simulink model "mrsMultiRobotAvoidance"  (R2019b)
settings: Solver=FixedStepAuto  StartTime=0.0  StopTime=inf  FixedStep=sampleTime  RelTol=1e-3
PreLoadFcn:
  | % Simulation parameters
  | load exampleMap
  | sampleTime = 0.05;
  | 
  | % Robot parameters
  | wheelRadius = 0.025;
  | robotRadius = 0.35;
  | 
  | % Lidar parameters
  | sensorOffset = [0,0];
  | scanAngles = linspace(-pi/2,pi/2,9)';
  | maxRange = 5;
libraries: mobileRoboticsLib x4
settings Model: EnablePacing=on  Creator=scastro  LastModifiedBy=jayas
settings DataIOCC: ReturnWorkspaceOutputs=off
settings DebuggingCC: PregeneratedLibrarySubsystemCodeDiagnostic=none  ArithmeticOperatorsInVariantConditions=warning
settings SFSimCC: SimUseLocalCustomCode=off  CustomCodeUndefinedFunction=UseInterfaceOnly
settings RTWCC: RTWUseLocalCustomCode=off

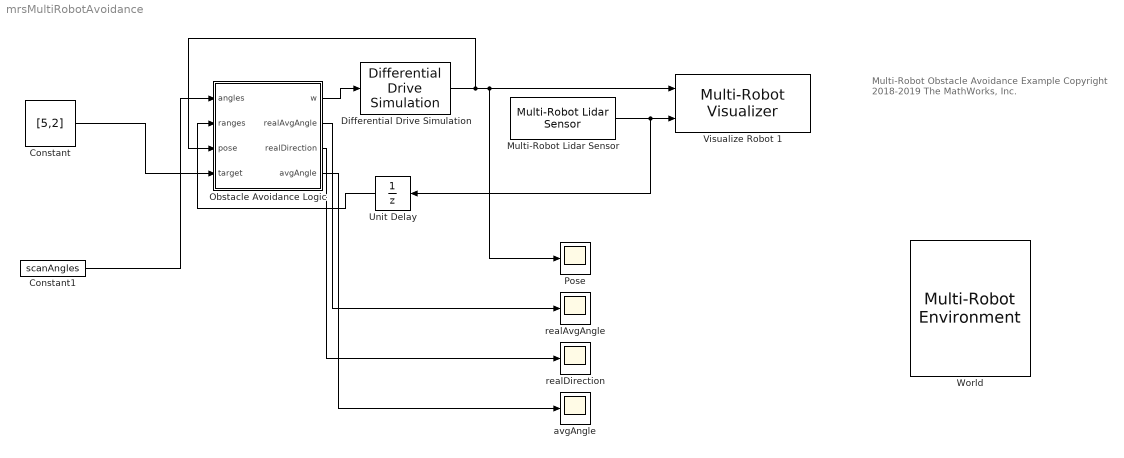
== system mrsMultiRobotAvoidance ==
  note: Multi-Robot Obstacle
      | Avoidance Example
      |
      | Copyright 2018-2019 The MathWorks, Inc.
  Constant : Constant  Value=[5,2]
  Constant1 : Constant  Value=scanAngles
  Differential Drive Simulation : mobileRoboticsLib/Kinematic Models/Differential Drive/Differential Drive Simulation  wheelRadius=wheelRadius  wheelBase=robotRadius  initX=10  initY=10  initAngle=0  Ts=sampleTime
      settings: SourceProductName=Mobile Robotics Simulation Toolbox
  Multi-Robot Lidar Sensor : mobileRoboticsLib/Environments/Multi-Robot Lidar Sensor  robotIdx=1  mapName=map  sensorOffset=sensorOffset  scanAngles=scanAngles  maxRange=maxRange
      settings: SourceProductName=Mobile Robotics Simulation Toolbox
  Obstacle Avoidance Logic : Stateflow chart  TreatAsAtomicUnit=on
  Pose : Scope
  Unit Delay : UnitDelay  SampleTime=-1  HasFrameUpgradeWarning=on
  Visualize Robot 1 : mobileRoboticsLib/Environments/Multi-Robot Visualizer  idx=1  radius=robotRadius  robotColor=[0 0 1]  showTraj=off  hasLidar=on  sensorOffset=sensorOffset  scanAngles=scanAngles  maxNumScans=0  hasObjDetector=off  objDetectorOffset=[0,0]  objDetectorAngle=0  objDetectorFOV=pi/2  objDetectorMaxRange=5  hasRobotDetector=off  robotDetectorOffset=[0,0]  robotDetectorAngle=0  robotDetectorFOV=pi/3  robotDetectorMaxRange=5  robotDetectorNumDetections=0
      settings: SourceProductName=Mobile Robotics Simulation Toolbox
  World : mobileRoboticsLib/Environments/Multi-Robot Environment  numRobots=1  mapName=map  showWaypoints=off  showObjects=off  objectColors=[1 0 0;0 1 0;0 0 1]  objectMarkers='s'  showRobotIds=on  plotSensorLines=on
      settings: SourceProductName=Mobile Robotics Simulation Toolbox
  avgAngle : Scope
  realAvgAngle : Scope
  realDirection : Scope
  wires:
  Differential Drive Simulation/1 -> Obstacle Avoidance Logic/3(pose), Pose/1, Visualize Robot 1/1
  Obstacle Avoidance Logic/1(w) -> Differential Drive Simulation/1
  Unit Delay/1 -> Obstacle Avoidance Logic/2(ranges)
  Constant1/1 -> Obstacle Avoidance Logic/1(angles)
  Multi-Robot Lidar Sensor/1 -> Unit Delay/1, Visualize Robot 1/2
  Constant/1 -> Obstacle Avoidance Logic/4(target)
  Obstacle Avoidance Logic/2(realAvgAngle) -> realAvgAngle/1
  Obstacle Avoidance Logic/3(realDirection) -> realDirection/1
  Obstacle Avoidance Logic/4(avgAngle) -> avgAngle/1

== stateflow chart mrsMultiRobotAvoidance/Obstacle Avoidance Logic ==
  state MainState [parallel]
    en,du:
    validIdx = ~isnan(ranges);
    validRanges = ranges(validIdx);
    validAngles = angles(validIdx);
    settings: executionOrder=1
    state Turn
      en,du:
      avgAngle = mean(validAngles./validRanges);
      realAvgAngle = CalculateStuff(pose, target, avgAngle);
      state Left
        en, du:
        w = [-12.5;12.5];
      state Right
        en, du:
        w = [12.5;-12.5];
      (default) -> (junction 39)
      (junction 39) -> Left [order 1] : [realAvgAngle < 0]
      (junction 39) -> (junction 43) [order 2]
      Left -> Right : [after(1,sec) && ...
          | realAvgAngle > 0]
      Right -> Left : [after(1,sec) && ...
          | realAvgAngle < 0]
      (junction 43) -> Right
    state GoStraight
      en:
      w = [25; 25];
    (default) -> GoStraight
    GoStraight -> Turn : [any(validRanges<=1)]
    Turn -> GoStraight : [all(validRanges>1)]
  data: posex function_input; targetx function_input; fn function_output; avgAnglex function_input; angles input; w output; ranges input; validRanges local size=numel(scanAngles); validIdx local; validAngles local size=numel(scanAngles); pose input; target input; x1 local; x2 local; y1 local; y2 local; realAvgAngle output; realDirection output; avgAngle output
  function fn =  CalculateStuff(posex, targetx, avgAnglex):
    | function fn =  CalculateStuff(posex, targetx, avgAnglex)
    |     x1 = posex(1);
    |     x2 = targetx(1);
    |     y1 = posex(2);
    |     y2 = targetx(2);
    |     realDirection = atan((y2-y1)/(x2-x1)) - posex(3);
    |     %fn = (avgAnglex + 2*realDirection)/3;
    |     fn = (avgAnglex*0 + 1*realDirection)/1;
    | end
